simulink model "Detailed_Comprehensive_Control_System_Project_Proposal"  (R2023a)
settings: Solver=FixedStepAuto  StartTime=0.0  StopTime=20  FixedStep=0.001  RelTol=1e-3  EnableMultiTasking=on
undefined symbols (not defined in the file or in its folder): DiscIntNeverNeededParam
libraries: arduinolib x8
settings Model: ExtModeTrigDuration=2  Creator=Mohamed Ezzelrgal  LastModifiedBy=Mohamed Ezzelrgal
settings OptimizationCC: EnhancedBackFolding=on  PassReuseOutputArgsAs=Individual arguments  ZeroExternalMemoryAtStartup=off  ZeroInternalMemoryAtStartup=off  MaxStackSize=64  OptimizeBlockOrder=speed  DifferentSizesBufferReuse=on  OptimizationCustomize=off  EfficientTunableParamExpr=on
settings DebuggingCC: ParameterTunabilityLossMsg=error
settings HardwareCC: ProdBitPerInt=16  ProdBitPerPointer=16  ProdBitPerSizeT=16  ProdBitPerPtrDiffT=16  ProdLargestAtomicFloat=None  ProdWordSize=8  ProdHWDeviceType=Atmel->AVR
settings SFSimCC: MATLABDynamicMemAlloc=off
settings RTWCC: Description=Embedded Coder  SystemTargetFile=ert.tlc  HardwareBoard=Arduino Uno  TemplateMakefile=ert_default_tmf  Toolchain=Arduino AVR  BuildConfiguration=Faster Runs
settings CodeAppCC: ForceParamTrailComments=on  IgnoreCustomStorageClasses=off  OperatorAnnotations=on  SimulinkDataObjDesc=on  SFDataObjDesc=on  InsertBlockDesc=on
settings ERTTargetCC: SupportContinuousTime=on  SupportVariableSizeSignals=on  ExtModeTransport=3  ExtModeStaticAlloc=on  ExtModeAutomaticAllocSize=off  ExtModeStaticAllocSize=250  ExtModeMexFile=ext_xcp  ExtModeIntrfLevel=Level2 - Open

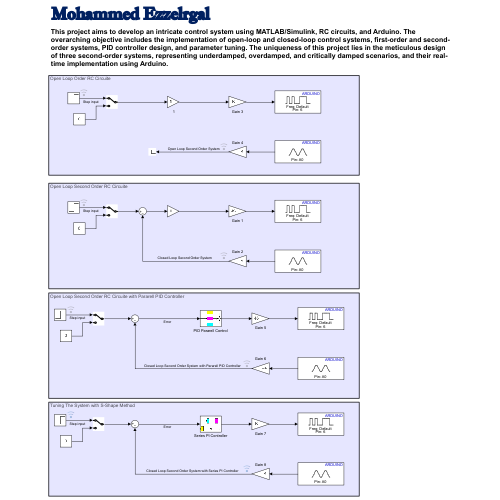
[thumbnail: Simulink's stored preview of the top-level diagram]
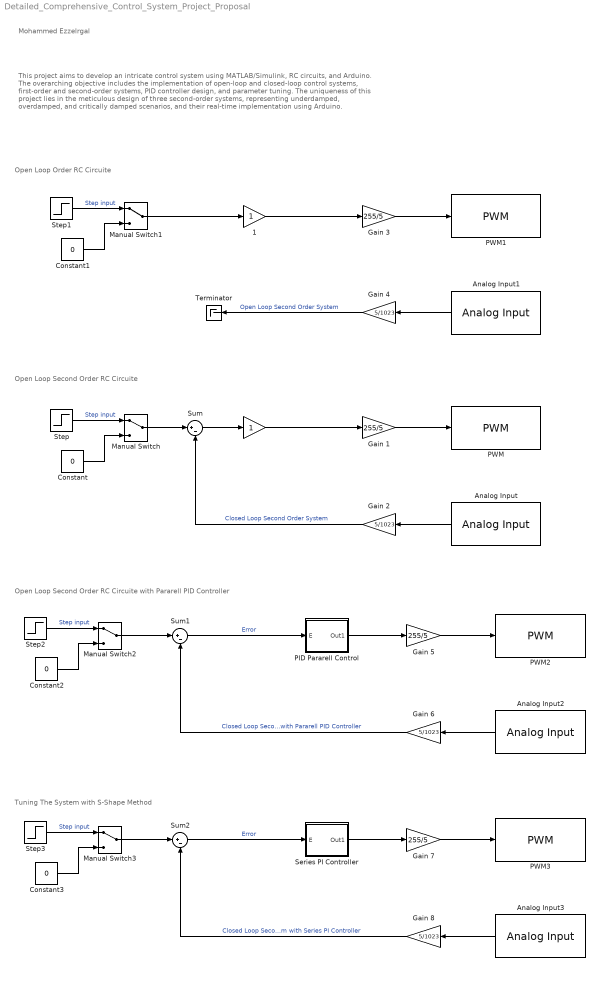
== system Detailed_Comprehensive_Control_System_Project_Proposal ==
  note: Tuning The System with S-Shape Method
  note: Open Loop Second Order RC Circuite with Pararell PID Controller
  note: Open Loop Second Order RC Circuite
  note: Open Loop Order RC Circuite
  note: This project aims to develop an intricate control system using MATLAB/Simulink, RC circuits, and Arduino. The overarching objective includes the implementation of open-loop and closed-loop control systems, first-order and second-order systems, PID controller design, and parameter tuning. The uniqueness of this project lies in the meticulous design of three second-order systems, representing underdamped, overdamped, and critically damped scenarios, and their real-time implementation using Arduino.
  note: Mohammed Ezzelrgal
  " " : Gain
  " 1" : Gain
  Analog Input{,1..3} (4 alike) : arduinolib/Analog Input  pinNumber=0  ReadResultsOnly=off  ConversionTriggerSource=Software  ExternalTriggerType=uint32( 0 )  OutputDataType=uint16  EnableConversionCompleteNotify=off  EnableOuputStatus=off  SampleTime=-1  blockPlatform=arduino
  Constant{,1..3} (4 alike) : Constant  Value=0
  Gain {1,3,5,7} (4 alike) : Gain  Gain=255/5
  Gain {2,4,6,8} (4 alike) : Gain  Gain=5/1023
  Manual Switch{,1..3} (4 alike) : ManualSwitch
  PID Pararell Control : Subsystem
      mask Display: image('C:\Users\User\Pictures\Screenshots\Screenshot 2024-04-04 033959.png'); % Use "Edit Image" on toolstrip to change.
  PWM{,1..3} (4 alike) : arduinolib/PWM  pinNumber=6  frequencyType=Default  desiredFrequency=490.2  achievableFrequency=490.2
  Series PI Controller : Subsystem
      mask Display: image('C:\Users\User\Pictures\Screenshots\Screenshot 2024-04-04 033454.png'); % Use "Edit Image" on toolstrip to change.
  Step{,1..3} (4 alike) : Step  SampleTime=0
  Sum : Sum  Inputs=|+-
  Sum1 : Sum  Inputs=|+-
  Sum2 : Sum  Inputs=|+-
  Terminator : Terminator
  wires:
  Step/1 -> Manual Switch/1  "Step input"
  Constant/1 -> Manual Switch/2
  " "/1 -> Gain 1/1
  Gain 1/1 -> PWM/1
  Analog Input/1 -> Gain 2/1
  Gain 2/1 -> Sum/2  "Closed Loop Second Order System"
  Manual Switch/1 -> Sum/1
  Sum/1 -> " "/1
  Manual Switch1/1 -> " 1"/1
  Analog Input1/1 -> Gain 4/1
  Gain 3/1 -> PWM1/1
  " 1"/1 -> Gain 3/1
  Constant1/1 -> Manual Switch1/2
  Step1/1 -> Manual Switch1/1  "Step input"
  Gain 4/1 -> Terminator/1  "Open Loop Second Order System"
  Manual Switch2/1 -> Sum1/1
  Gain 6/1 -> Sum1/2  "Closed Loop Second Order System with Pararell PID Controller"
  Analog Input2/1 -> Gain 6/1
  Gain 5/1 -> PWM2/1
  Constant2/1 -> Manual Switch2/2
  Step2/1 -> Manual Switch2/1  "Step input"
  Sum1/1 -> PID Pararell Control/1(E)  "Error"
  PID Pararell Control/1(Out1) -> Gain 5/1
  Series PI Controller/1(Out1) -> Gain 7/1
  Sum2/1 -> Series PI Controller/1(E)  "Error"
  Step3/1 -> Manual Switch3/1  "Step input"
  Constant3/1 -> Manual Switch3/2
  Gain 7/1 -> PWM3/1
  Analog Input3/1 -> Gain 8/1
  Gain 8/1 -> Sum2/2  "Closed Loop Second Order System with Series PI Controller"
  Manual Switch3/1 -> Sum2/1

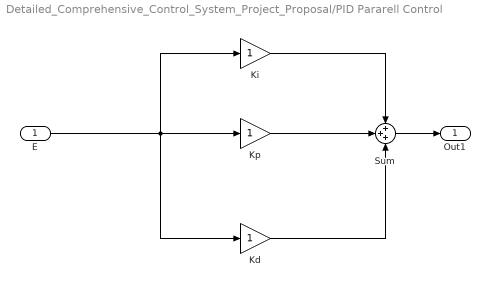
== system Detailed_Comprehensive_Control_System_Project_Proposal/PID Pararell Control ==
  E : Inport
  Kd : Gain
  Ki : Gain
  Kp : Gain
  Sum : Sum  Inputs=+++
  Out1 : Outport
  wires:
  E/1 -> Kp/1, Ki/1, Kd/1
  Sum/1 -> Out1/1
  Kp/1 -> Sum/2
  Ki/1 -> Sum/1
  Kd/1 -> Sum/3

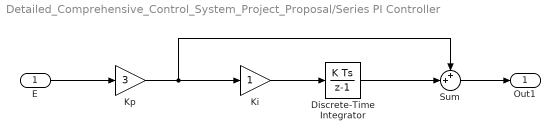
== system Detailed_Comprehensive_Control_System_Project_Proposal/Series PI Controller ==
  E : Inport
  Discrete-Time Integrator : DiscreteIntegrator  SampleTime=-1  ICPrevOutput=DiscIntNeverNeededParam  ICPrevScaledInput=DiscIntNeverNeededParam
  Ki : Gain
  Kp : Gain  Gain=3
  Sum : Sum  Inputs=++|
  Out1 : Outport
  wires:
  Sum/1 -> Out1/1
  E/1 -> Kp/1
  Ki/1 -> Discrete-Time Integrator/1
  Kp/1 -> Sum/1, Ki/1
  Discrete-Time Integrator/1 -> Sum/2
